simulink model "CurrentSensor_sim_2020"  (R2020b)
settings: Solver=ode4  StartTime=0.0  StopTime=2  FixedStep=0.05  RelTol=1e-3
settings Model: Creator=005274  LastModifiedBy=005274

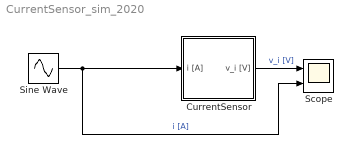
== system CurrentSensor_sim_2020 ==
  CurrentSensor : Subsystem  mask(CurrentSensorModel){}
  Scope : Scope  NumInputPorts=2
  Sine Wave : Sin  Amplitude=25  Frequency=2*pi  SampleTime=0
  wires:
  CurrentSensor/1(v_i [V]) -> Scope/1  "v_i [V]"
  Sine Wave/1 -> CurrentSensor/1(i [A]), Scope/2  "i [A]"

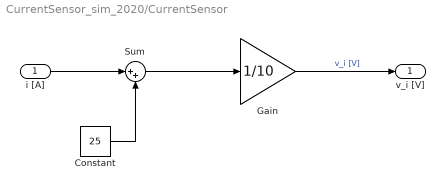
== system CurrentSensor_sim_2020/CurrentSensor ==
  i [A] : Inport
  Constant : Constant  Value=25
  Gain : Gain  Gain=1/10
  Sum : Sum  Inputs=|++
  v_i [V] : Outport
  wires:
  Sum/1 -> Gain/1
  Constant/1 -> Sum/2
  Gain/1 -> v_i [V]/1  "v_i [V]"
  i [A]/1 -> Sum/1
